simulink model "ThreePhaseInverter"  (R2025a)
settings: Solver=VariableStepAuto  StartTime=0.0  StopTime=0.2  RelTol=1e-3
libraries: spsDiodeLib x6, spsMosfetLib x6, spsSeriesRLCBranchLib x3, spsVoltageMeasurementLib x2, spsCurrentMeasurementLib x1, spsDCVoltageSourceLib x1, spsTriangleGeneratorLib x1, sps_lib x1
settings Model: Creator=aditl  LastModifiedBy=aditl

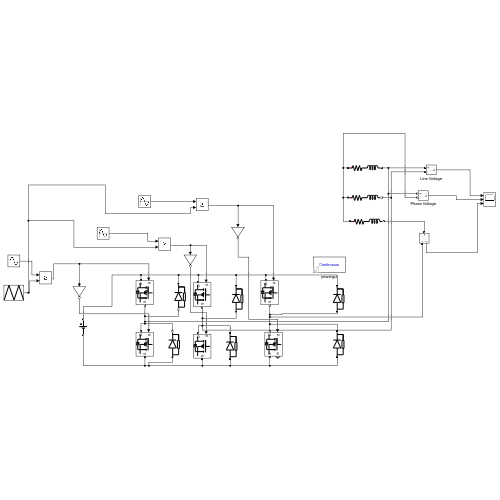
[thumbnail: Simulink's stored preview of the top-level diagram]
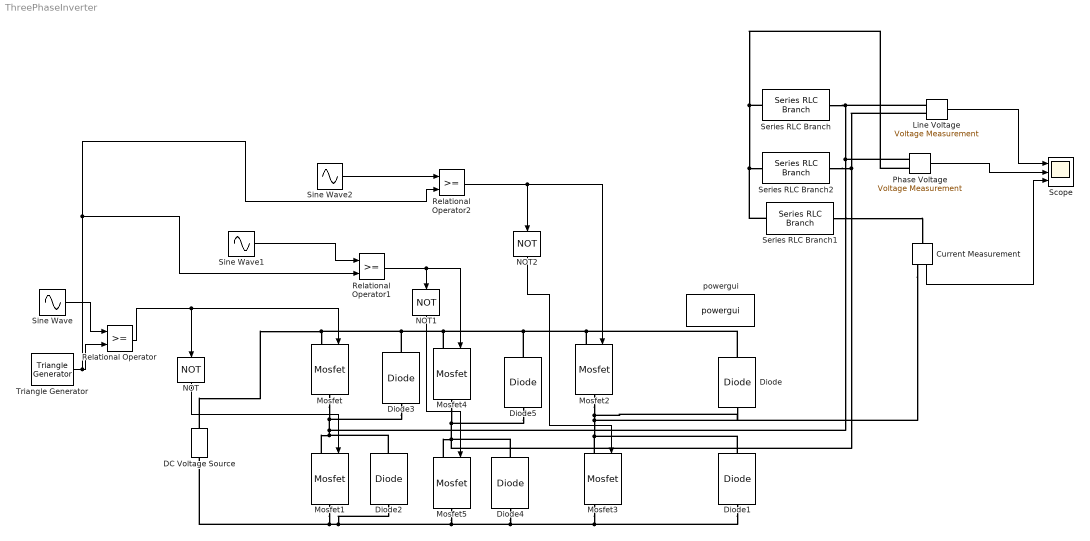
== system ThreePhaseInverter ==
  Current Measurement : spsCurrentMeasurementLib/Current Measurement  PhasorSimulation=off  OutputType=Complex  PSBequivalent=0
  DC Voltage Source : spsDCVoltageSourceLib/DC Voltage Source  Amplitude=100  Measurements=None
  Diode{,1..5} (6 alike) : spsDiodeLib/Diode  Ron=0.001  Lon=0  Vf=0.8  IC=0  UseSnubber=0  Rs=500  Cs=250e-9  Measurements=off
  Line Voltage : spsVoltageMeasurementLib/Voltage Measurement  PhasorSimulation=off  OutputType=Complex  PSBequivalent=0
  Mosfet{,1..2,4..5} (5 alike) : spsMosfetLib/Mosfet  Ron=0.1  Lon=0  Rd=0.01  Vfd=0  IC=0  Rs=1e5  Cs=inf  Measurements=off
  Mosfet3 : spsMosfetLib/Mosfet  Ron=0.1  Lon=0  Rd=0.01  Vfd=0  IC=0  Rs=1e5  Cs=inf  Measurements=on
  NOT : Logic  Operator=NOT  IconShape=distinctive  AllPortsSameDT=off  OutDataTypeStr=boolean
  NOT1 : Logic  Operator=NOT  IconShape=distinctive  AllPortsSameDT=off  OutDataTypeStr=boolean
  NOT2 : Logic  Operator=NOT  IconShape=distinctive  AllPortsSameDT=off  OutDataTypeStr=boolean
  Phase Voltage : spsVoltageMeasurementLib/Voltage Measurement  PhasorSimulation=off  OutputType=Complex  PSBequivalent=0
  Relational Operator : RelationalOperator  OutDataTypeStr=boolean  RndMeth=Simplest  InputSameDT=off
  Relational Operator1 : RelationalOperator  OutDataTypeStr=boolean  RndMeth=Simplest  InputSameDT=off
  Relational Operator2 : RelationalOperator  OutDataTypeStr=boolean  RndMeth=Simplest  InputSameDT=off
  Scope : Scope  NumInputPorts=3
      settings: ActiveDisplayYMinimum=-124.95561  ActiveDisplayYMaximum=124.95573
  Series RLC Branch : spsSeriesRLCBranchLib/Series RLC Branch  LConnTagsString=__new0  RConnTagsString=__new0  BranchType=RL  Resistance=25  Inductance=1e-3  SetiL0=off  InitialCurrent=0  Capacitance=1e-6  Setx0=off  InitialVoltage=0  Measurements=None
  Series RLC Branch1 : spsSeriesRLCBranchLib/Series RLC Branch  LConnTagsString=__new0  RConnTagsString=__new0  BranchType=RL  Resistance=25  Inductance=1e-3  SetiL0=off  InitialCurrent=0  Capacitance=1e-6  Setx0=off  InitialVoltage=0  Measurements=None
  Series RLC Branch2 : spsSeriesRLCBranchLib/Series RLC Branch  LConnTagsString=__new0  RConnTagsString=__new0  BranchType=RL  Resistance=25  Inductance=1e-3  SetiL0=off  InitialCurrent=0  Capacitance=1e-6  Setx0=off  InitialVoltage=0  Measurements=None
  Sine Wave : Sin  Amplitude=1.2  Frequency=50*2*pi  SampleTime=0
  Sine Wave1 : Sin  Amplitude=1.2  Frequency=50*2*pi  Phase=120*(pi/180)  SampleTime=0
  Sine Wave2 : Sin  Amplitude=1.2  Frequency=50*2*pi  Phase=-120*(pi/180)  SampleTime=0
  Triangle Generator : spsTriangleGeneratorLib/Triangle Generator  Freq=5000  Phase=0  Ts=0
  powergui : sps_lib/powergui  Priority=1  SimulationMode=Continuous  SampleTime=50e-6  frequency=60  Iterations=50  frequencyindice=0  Pbase=100e6  ErrMax=1e-4  UnitsV=kV  UnitsW=MW  buscounter=0  FunctionMessages=off  echomessages=off  EnableUseOfTLC=off  CurrentSourceSwitches=off  DisableSnubberDevices=off  DisableRonSwitches=off  DisableVfSwitches=off  DisplayEquations=off  AutomaticDiscreteSolvers=off  SolverType=Tustin/Backward Euler (TBE)  Interpol=off  ExternalGateDelay=off  methode=off  Ts=100  x0status=blocks  SPID=on  SwTol=0  HookPort=off  NonlinearTolerance=1e-4  nMaxIteration=100  ContinueOnMaxIteration=off  RestoreLinks=warning  ResistiveCurrentMeasurement=off  Frange=[0:2:500]  Ylog=off  Xlog=on  ShowGrid=off  save=off  variable=ZData  structure=0  ZoomFFT=off  StartTime=0.0  cycles=1  DisplayStyle=1  fundamental=60  FreqAxis=off  MaxFrequency=1000  frequencyindicesteady=1  RmsSteady=1  display=off
  wires:
  Sine Wave/1 -> Relational Operator/1
  Triangle Generator/1 -> Relational Operator2/2, Relational Operator1/2, Relational Operator/2
  Relational Operator/1 -> NOT/1, Mosfet/1
  NOT/1 -> Mosfet1/1
  Sine Wave1/1 -> Relational Operator1/1
  Relational Operator1/1 -> NOT1/1, Mosfet4/1
  NOT1/1 -> Mosfet5/1
  Sine Wave2/1 -> Relational Operator2/1
  Relational Operator2/1 -> NOT2/1, Mosfet2/1
  NOT2/1 -> Mosfet3/1
  Current Measurement/1 -> Scope/3
  Phase Voltage/1 -> Scope/2
  Line Voltage/1 -> Scope/1
  connections:
  Mosfet1/LConn1 -- Diode2/RConn1 -- Series RLC Branch/RConn1 -- Line Voltage/LConn1 -- Phase Voltage/LConn1 -- Mosfet/RConn1 -- Diode3/LConn1
  Diode1/LConn1 -- Mosfet3/RConn1 -- Diode4/LConn1 -- Mosfet5/RConn1 -- Diode2/LConn1 -- Mosfet1/RConn1 -- DC Voltage Source/LConn1
  Mosfet/LConn1 -- DC Voltage Source/RConn1 -- Diode5/RConn1 -- Diode/RConn1 -- Mosfet2/LConn1 -- Mosfet4/LConn1 -- Diode3/RConn1
  Diode/LConn1 -- Mosfet2/RConn1 -- Current Measurement/RConn1 -- Mosfet3/LConn1 -- Diode1/RConn1
  Diode5/LConn1 -- Mosfet4/RConn1 -- Line Voltage/LConn2 -- Series RLC Branch2/RConn1 -- Diode4/RConn1 -- Mosfet5/LConn1
  Series RLC Branch/LConn1 -- Series RLC Branch1/LConn1 -- Series RLC Branch2/LConn1 -- Phase Voltage/LConn2
  Series RLC Branch1/RConn1 -- Current Measurement/LConn1
